simulink model "NonLin_MagLev"  (Simulink 10.3)
settings: Solver=ode4  StartTime=0.0  StopTime=20  FixedStep=0.005  RelTol=1e-3  EnableMultiTasking=on
undefined symbols (not defined in the file or in its folder): Kd, Ki, Kp, magnitude
settings Model: Creator=AMM  LastModifiedBy=ABRAM  MultithreadedSim=on
settings SolverCC: AutoInsertRateTranBlk=on
settings DataIOCC: LimitDataPoints=on
settings DebuggingCC: SolverPrmCheckMsg=warning

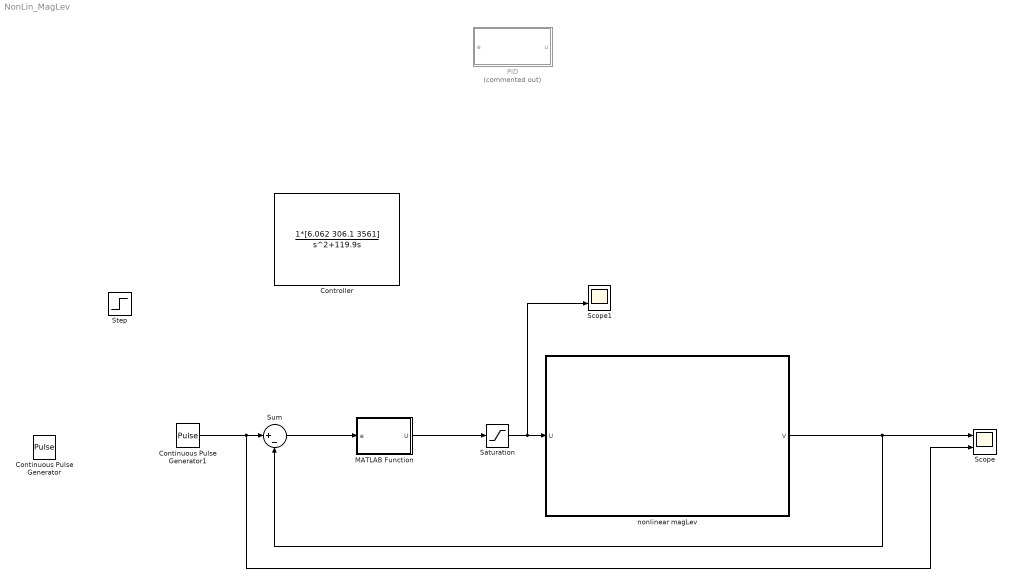
== system NonLin_MagLev ==
  Continuous Pulse Generator : DiscretePulseGenerator  PulseType=Time based  Period=1  PulseWidth=50
  Continuous Pulse Generator1 : DiscretePulseGenerator  PulseType=Time based  Period=3  PulseWidth=50
  "Controller " : TransferFcn  Numerator=1*[6.062 306.1 3561]  Denominator=[1.0000 119.9 0]
  MATLAB Function : MATLAB Function  TreatAsAtomicUnit=on
  PID : Subsystem  Commented=on
  Saturation : Saturate  UpperLimit=5  LowerLimit=-5
  Scope : Scope  NumInputPorts=2
  Scope1 : Scope  NumInputPorts=2
  Step : Step  SampleTime=0
  Sum : Sum  Inputs=|+-
  "nonlinear magLev " : Subsystem
  wires:
  Continuous Pulse Generator1/1 -> Scope/2, Sum/1
  "nonlinear magLev "/1(V) -> Sum/2, Scope/1
  Saturation/1 -> "nonlinear magLev "/1(U), Scope1/2
  Sum/1 -> MATLAB Function/1(e)
  MATLAB Function/1(U) -> Saturation/1

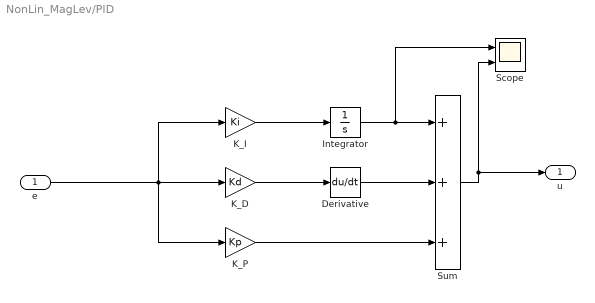
== system NonLin_MagLev/PID ==
  e : Inport
  Derivative : Derivative
  Integrator : Integrator  LimitOutput=on  UpperSaturationLimit=3  LowerSaturationLimit=-3
  K_D : Gain  Gain=Kd
  K_I : Gain  Gain=Ki
  "K_P " : Gain  Gain=Kp
  Scope : Scope  NumInputPorts=2
  Sum : Sum  Inputs=+++
  u : Outport  VectorParamsAs1DForOutWhenUnconnected=off
  wires:
  Sum/1 -> Scope/2, u/1
  Integrator/1 -> Sum/1, Scope/1
  K_I/1 -> Integrator/1
  Derivative/1 -> Sum/2
  K_D/1 -> Derivative/1
  "K_P "/1 -> Sum/3
  e/1 -> "K_P "/1, K_I/1, K_D/1

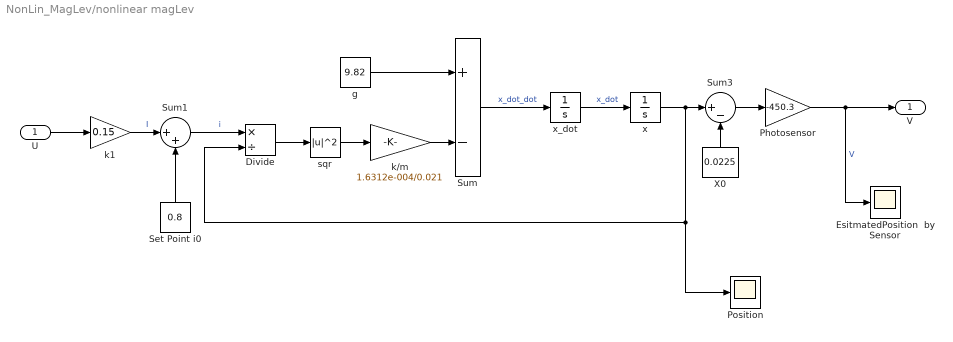
== system NonLin_MagLev/nonlinear magLev  ==
  U : Inport
  Divide : Product  Inputs=*/
  EsitmatedPosition  by Sensor : Scope
  Photosensor : Gain  Gain=-450.3
  Position : Scope
  Set Point i0 : Constant  Value=0.8
  Sum : Sum  Inputs=+-
  Sum1 : Sum  Inputs=|++
  Sum3 : Sum  Inputs=|+-
  X0 : Constant  Value=0.0225
  g : Constant  Value=9.82
  k/m : Gain  Gain=1.6312e-004/0.021
  k1 : Gain  Gain=0.15
  sqr : Math  Operator=magnitude^2  SignedPower=on  SaturateOnIntegerOverflow=on
  x : Integrator  InitialCondition=0.0225  LimitOutput=on  UpperSaturationLimit=0.027  LowerSaturationLimit=0.018  ContinuousStateAttributes='x'
  x_dot : Integrator  ContinuousStateAttributes='x_dot'
  V : Outport  VectorParamsAs1DForOutWhenUnconnected=off
  wires:
  x/1 -> Sum3/1, Position/1, Divide/2
  Photosensor/1 -> V/1, EsitmatedPosition  by Sensor/1  "V"
  g/1 -> Sum/1
  Sum1/1 -> Divide/1  "i"
  k/m/1 -> Sum/2
  x_dot/1 -> x/1  "x_dot"
  Divide/1 -> sqr/1
  Sum/1 -> x_dot/1  "x_dot_dot"
  Sum3/1 -> Photosensor/1
  k1/1 -> Sum1/1  "I"
  Set Point i0/1 -> Sum1/2
  X0/1 -> Sum3/2
  sqr/1 -> k/m/1
  U/1 -> k1/1

== matlab function MATLAB Function ==
  settings: updateMethod=DISCRETE  sampleTime=0.005
  data: e input double; U output double
function U = fcn(e)

persistent e_prev I_u

if (isempty(e_prev))
    e_prev=0;
end
if (isempty(I_u))
    I_u=0;
end

kp = 1.1543;
ki = 2.1241;
kd = 0.0368;
Ts=0.005;
Isat=3;

I_u=I_u + ki*e*Ts;

if  Isat> 0.0
    if I_u >Isat
        I_u =Isat;
    end
    if I_u <-Isat
        I_u =-Isat;
    end
end

U = kp*e + I_u + kd *(e - e_prev) / Ts;
e_prev=e;

if (U >5)
    U=5;  
end
if (U <-5)
    U=-5;
end
end
